simulink model "TomaDatosPrimerOrdenRuido_ver2017a"  (R2017a)
settings: Solver=ode45  StartTime=0.0  StopTime=10.0  RelTol=1e-3
libraries: simulink x1
settings Model: Creator=Jesus  LastModifiedBy=jesus
settings DataIOCC: LimitDataPoints=on  SaveFormat=Array
settings OptimizationCC: BlockReduction=off  BooleanDataType=off  LifeSpan=inf
settings DebuggingCC: SaveWithParameterizedLinksMsg=none  UnderspecifiedInitializationDetection=Classic  MergeDetectMultiDrivingBlocksExec=none  SignalResolutionControl=TryResolveAllWithWarning  SFUnexpectedBacktrackingDiag=warning  SFNoUnconditionalDefaultTransitionDiag=warning  SFExecutionAtInitializationDiag=none
settings HardwareCC: ProdBitPerPointer=32  ProdBitPerSizeT=32  ProdBitPerPtrDiffT=32  ProdLargestAtomicFloat=None  ProdIntDivRoundTo=Undefined  ProdEndianess=Unspecified  ProdWordSize=32  ProdHWDeviceType=32-bit Generic  TargetUnknown=on
settings ModelReferenceCC: PropagateSignalLabelsOutOfModel=off
settings GRTTargetCC: TargetLangStandard=C89/C90 (ANSI)  GeneratePreprocessorConditionals=Disable all
settings ConfigComp: CovMetricSettings=dw  CovHtmlReporting=on  CovSaveCumulativeToWorkspaceVar=on  CovSaveSingleToWorkspaceVar=on  CovExternalEMLEnable=off  CovSFcnEnable=off

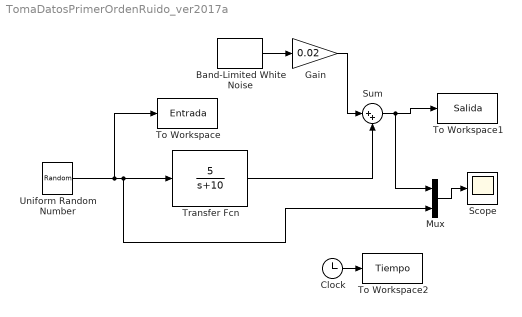
== system TomaDatosPrimerOrdenRuido_ver2017a ==
  Band-Limited White Noise : simulink/Sources/Band-Limited White Noise  Cov=[0.1]  Ts=0.01  seed=[23341]
  Clock : Clock
  Gain : Gain  Gain=0.02
  Mux : Mux  Inputs=2
  Scope : Scope
  Sum : Sum  Inputs=|++
  To Workspace : ToWorkspace  VariableName=Entrada  SampleTime=0.01
  To Workspace1 : ToWorkspace  VariableName=Salida  SampleTime=0.01
  To Workspace2 : ToWorkspace  VariableName=Tiempo  SampleTime=0.01
  Transfer Fcn : TransferFcn  Numerator=[5]  Denominator=[1 10]
  Uniform Random Number : UniformRandomNumber  Minimum=0  Maximum=5  SampleTime=0.6
  wires:
  Uniform Random Number/1 -> To Workspace/1, Mux/2, Transfer Fcn/1
  Mux/1 -> Scope/1
  Clock/1 -> To Workspace2/1
  Transfer Fcn/1 -> Sum/2
  Sum/1 -> Mux/1, To Workspace1/1
  Band-Limited White Noise/1 -> Gain/1
  Gain/1 -> Sum/1
